simulink model "case2"  (R2024b)
settings: Solver=FixedStepAuto  StartTime=0  StopTime=1  FixedStep=1e-7  RelTol=1e-3
values from neighbouring files (symbols this model uses):
  SG_D_1_D = 0.01056    [IEEE9_case_parameters.m]    (also in case1_parameters.m; case2_parameters.m; case3_parameters.m; case4_parameters.m)
  SG_D_1_EnableSaturation = 0    [IEEE9_case_parameters.m]    (also in case1_parameters.m; case2_parameters.m; case3_parameters.m; case4_parameters.m)
  SG_D_1_f0 = 60    [IEEE9_case_parameters.m]    (also in case1_parameters.m; case2_parameters.m; case3_parameters.m; case4_parameters.m)
  SG_D_1_H = 7.5    [IEEE9_case_parameters.m]    (also in case1_parameters.m; case2_parameters.m; case3_parameters.m; case4_parameters.m)
  SG_D_1_K_A = 20    [IEEE9_case_parameters.m]    (also in case1_parameters.m; case2_parameters.m; case3_parameters.m; case4_parameters.m)
  SG_D_1_K_E = 1.000000e+1    (= 10)    [IEEE9_case_parameters.m]    (also in case1_parameters.m; case2_parameters.m; case3_parameters.m; case4_parameters.m)
  SG_D_1_K_F = 2.363    [IEEE9_case_parameters.m]    (also in case1_parameters.m; case2_parameters.m; case3_parameters.m; case4_parameters.m)
  SG_D_1_K_s = 0.5    [IEEE9_case_parameters.m]    (also in case1_parameters.m = 5; case2_parameters.m = 5; case3_parameters.m = 5; case4_parameters.m = 5)
  SG_D_1_R_a = 0.001088    [IEEE9_case_parameters.m]    (also in case1_parameters.m; case2_parameters.m; case3_parameters.m; case4_parameters.m)
  SG_D_1_S_A = 1    [IEEE9_case_parameters.m]    (also in case1_parameters.m; case2_parameters.m; case3_parameters.m; case4_parameters.m)
  SG_D_1_S_B = 0.103    [IEEE9_case_parameters.m]    (also in case1_parameters.m; case2_parameters.m; case3_parameters.m; case4_parameters.m)
  SG_D_1_S_N = 10.659857    [IEEE9_case_parameters.m]    (also in case1_parameters.m; case2_parameters.m; case3_parameters.m; case4_parameters.m)
  SG_D_1_SpeedPara = 200    [IEEE9_case_parameters.m]    (also in case1_parameters.m; case2_parameters.m; case3_parameters.m; case4_parameters.m)
  SG_D_1_T_0 = 0.720173    [IEEE9_case_parameters.m]    (also in case1_parameters.m = 0.755522; case2_parameters.m = 0.808931; case3_parameters.m = 0.869402; case4_parameters.m = 0.729316)
  SG_D_1_T_1 = 0.3    [IEEE9_case_parameters.m]    (also in case1_parameters.m; case2_parameters.m; case3_parameters.m; case4_parameters.m)
  SG_D_1_T_2 = 0.05    [IEEE9_case_parameters.m]    (also in case1_parameters.m; case2_parameters.m; case3_parameters.m; case4_parameters.m)
  SG_D_1_T_3 = 0.02    [IEEE9_case_parameters.m]    (also in case1_parameters.m; case2_parameters.m; case3_parameters.m; case4_parameters.m)
  SG_D_1_T_4 = 0.005    [IEEE9_case_parameters.m]    (also in case1_parameters.m; case2_parameters.m; case3_parameters.m; case4_parameters.m)
  SG_D_1_T_A = 0.02    [IEEE9_case_parameters.m]    (also in case1_parameters.m; case2_parameters.m; case3_parameters.m; case4_parameters.m)
  SG_D_1_T_dd = 8.000000e+0    (= 8)    [IEEE9_case_parameters.m]    (also in case1_parameters.m; case2_parameters.m; case3_parameters.m; case4_parameters.m)
  SG_D_1_T_ddd = 0.04    [IEEE9_case_parameters.m]    (also in case1_parameters.m; case2_parameters.m; case3_parameters.m; case4_parameters.m)
  SG_D_1_T_E = 0.314    [IEEE9_case_parameters.m]    (also in case1_parameters.m; case2_parameters.m; case3_parameters.m; case4_parameters.m)
  SG_D_1_T_F = 0.35    [IEEE9_case_parameters.m]    (also in case1_parameters.m; case2_parameters.m; case3_parameters.m; case4_parameters.m)
  SG_D_1_T_qd = 0.8    [IEEE9_case_parameters.m]    (also in case1_parameters.m; case2_parameters.m; case3_parameters.m; case4_parameters.m)
  SG_D_1_T_qdd = 0.02    [IEEE9_case_parameters.m]    (also in case1_parameters.m; case2_parameters.m; case3_parameters.m; case4_parameters.m)
  SG_D_1_T_speed = 0.1    [IEEE9_case_parameters.m]    (also in case1_parameters.m = 200; case2_parameters.m = 200; case3_parameters.m = 200; case4_parameters.m = 200)
  SG_D_1_T_w = 0.5    [IEEE9_case_parameters.m]    (also in case1_parameters.m; case2_parameters.m; case3_parameters.m; case4_parameters.m)
  SG_D_1_V_ref = 1.990276    [IEEE9_case_parameters.m]    (also in case1_parameters.m = 2.042296; case2_parameters.m = 2.051388; case3_parameters.m = 2.089584; case4_parameters.m = 2.01845)
  SG_D_1_w_ref = 376.991118    [IEEE9_case_parameters.m]    (also in case1_parameters.m; case2_parameters.m; case3_parameters.m; case4_parameters.m)
  SG_D_1_wb = 6.000000e+1    (= 60)    [IEEE9_case_parameters.m]    (also in case1_parameters.m; case2_parameters.m; case3_parameters.m; case4_parameters.m)
  SG_D_1_x_d = 1.9    [IEEE9_case_parameters.m]    (also in case1_parameters.m; case2_parameters.m; case3_parameters.m; case4_parameters.m)
  SG_D_1_x_dd = 0.302    [IEEE9_case_parameters.m]    (also in case1_parameters.m; case2_parameters.m; case3_parameters.m; case4_parameters.m)
  SG_D_1_x_ddd = 0.204    [IEEE9_case_parameters.m]    (also in case1_parameters.m; case2_parameters.m; case3_parameters.m; case4_parameters.m)
  SG_D_1_x_l = 0.05    [IEEE9_case_parameters.m]    (also in case1_parameters.m; case2_parameters.m; case3_parameters.m; case4_parameters.m)
  SG_D_1_x_q = 1.3    [IEEE9_case_parameters.m]    (also in case1_parameters.m; case2_parameters.m; case3_parameters.m; case4_parameters.m)
  SG_D_1_x_qd = 0.5    [IEEE9_case_parameters.m]    (also in case1_parameters.m; case2_parameters.m; case3_parameters.m; case4_parameters.m)
  SG_D_1_x_qdd = 0.3    [IEEE9_case_parameters.m]    (also in case1_parameters.m; case2_parameters.m; case3_parameters.m; case4_parameters.m)
  SG_D_2_D = 0.02    [IEEE9_case_parameters.m]    (also in case1_parameters.m; case2_parameters.m; case3_parameters.m; case4_parameters.m)
  SG_D_2_EnableSaturation = 0    [IEEE9_case_parameters.m]    (also in case1_parameters.m; case2_parameters.m; case3_parameters.m; case4_parameters.m)
  SG_D_2_f0 = 60    [IEEE9_case_parameters.m]    (also in case1_parameters.m; case2_parameters.m; case3_parameters.m; case4_parameters.m)
  SG_D_2_H = 8.000000e+0    (= 8)    [IEEE9_case_parameters.m]    (also in case1_parameters.m; case2_parameters.m; case3_parameters.m; case4_parameters.m)
  SG_D_2_K_A = 20    [IEEE9_case_parameters.m]    (also in case1_parameters.m; case2_parameters.m; case3_parameters.m; case4_parameters.m)
  SG_D_2_K_E = 1.000000e+1    (= 10)    [IEEE9_case_parameters.m]    (also in case1_parameters.m; case2_parameters.m; case3_parameters.m; case4_parameters.m)
  SG_D_2_K_F = 2.363    [IEEE9_case_parameters.m]    (also in case1_parameters.m; case2_parameters.m; case3_parameters.m; case4_parameters.m)
  SG_D_2_K_s = 0.5    [IEEE9_case_parameters.m]    (also in case1_parameters.m = 4; case2_parameters.m = 4; case3_parameters.m = 4; case4_parameters.m = 4)
  SG_D_2_R_a = 0.001088    [IEEE9_case_parameters.m]    (also in case1_parameters.m; case2_parameters.m; case3_parameters.m; case4_parameters.m)
  SG_D_2_S_A = 1    [IEEE9_case_parameters.m]    (also in case1_parameters.m; case2_parameters.m; case3_parameters.m; case4_parameters.m)
  SG_D_2_S_B = 0.103    [IEEE9_case_parameters.m]    (also in case1_parameters.m; case2_parameters.m; case3_parameters.m; case4_parameters.m)
  SG_D_2_S_N = 10.659857    [IEEE9_case_parameters.m]    (also in case1_parameters.m; case2_parameters.m; case3_parameters.m; case4_parameters.m)
  SG_D_2_SpeedPara = 200    [IEEE9_case_parameters.m]    (also in case1_parameters.m; case2_parameters.m; case3_parameters.m; case4_parameters.m)
  SG_D_2_T_0 = 1.632913    [IEEE9_case_parameters.m]    (also in case1_parameters.m = 1.632925; case2_parameters.m = 1.632915; case3_parameters.m = 1.632914; case4_parameters.m = 1.632927)
  SG_D_2_T_1 = 0.2    [IEEE9_case_parameters.m]    (also in case1_parameters.m; case2_parameters.m; case3_parameters.m; case4_parameters.m)
  SG_D_2_T_2 = 0.05    [IEEE9_case_parameters.m]    (also in case1_parameters.m; case2_parameters.m; case3_parameters.m; case4_parameters.m)
  SG_D_2_T_3 = 0.02    [IEEE9_case_parameters.m]    (also in case1_parameters.m; case2_parameters.m; case3_parameters.m; case4_parameters.m)
  SG_D_2_T_4 = 0.005    [IEEE9_case_parameters.m]    (also in case1_parameters.m; case2_parameters.m; case3_parameters.m; case4_parameters.m)
  SG_D_2_T_A = 0.02    [IEEE9_case_parameters.m]    (also in case1_parameters.m; case2_parameters.m; case3_parameters.m; case4_parameters.m)
  SG_D_2_T_dd = 7.9    [IEEE9_case_parameters.m]    (also in case1_parameters.m; case2_parameters.m; case3_parameters.m; case4_parameters.m)
  SG_D_2_T_ddd = 0.04    [IEEE9_case_parameters.m]    (also in case1_parameters.m; case2_parameters.m; case3_parameters.m; case4_parameters.m)
  SG_D_2_T_E = 0.314    [IEEE9_case_parameters.m]    (also in case1_parameters.m; case2_parameters.m; case3_parameters.m; case4_parameters.m)
  SG_D_2_T_F = 0.35    [IEEE9_case_parameters.m]    (also in case1_parameters.m; case2_parameters.m; case3_parameters.m; case4_parameters.m)
  SG_D_2_T_qd = 0.8    [IEEE9_case_parameters.m]    (also in case1_parameters.m; case2_parameters.m; case3_parameters.m; case4_parameters.m)
  SG_D_2_T_qdd = 0.015    [IEEE9_case_parameters.m]    (also in case1_parameters.m; case2_parameters.m; case3_parameters.m; case4_parameters.m)
  SG_D_2_T_speed = 0.1    [IEEE9_case_parameters.m]    (also in case1_parameters.m = 150; case2_parameters.m = 150; case3_parameters.m = 150; case4_parameters.m = 150)
  SG_D_2_T_w = 0.35    [IEEE9_case_parameters.m]    (also in case1_parameters.m; case2_parameters.m; case3_parameters.m; case4_parameters.m)
  SG_D_2_V_ref = 2.58547    [IEEE9_case_parameters.m]    (also in case1_parameters.m = 2.597896; case2_parameters.m = 2.587136; case3_parameters.m = 2.586042; case4_parameters.m = 2.599679)
  SG_D_2_w_ref = 376.991118    [IEEE9_case_parameters.m]    (also in case1_parameters.m; case2_parameters.m; case3_parameters.m; case4_parameters.m)
  SG_D_2_wb = 6.000000e+1    (= 60)    [IEEE9_case_parameters.m]    (also in case1_parameters.m; case2_parameters.m; case3_parameters.m; case4_parameters.m)
  SG_D_2_x_d = 1.8    [IEEE9_case_parameters.m]    (also in case1_parameters.m; case2_parameters.m; case3_parameters.m; case4_parameters.m)
  SG_D_2_x_dd = 0.302    [IEEE9_case_parameters.m]    (also in case1_parameters.m; case2_parameters.m; case3_parameters.m; case4_parameters.m)
  SG_D_2_x_ddd = 0.204    [IEEE9_case_parameters.m]    (also in case1_parameters.m; case2_parameters.m; case3_parameters.m; case4_parameters.m)
  SG_D_2_x_l = 0.05    [IEEE9_case_parameters.m]    (also in case1_parameters.m; case2_parameters.m; case3_parameters.m; case4_parameters.m)
  SG_D_2_x_q = 1.25    [IEEE9_case_parameters.m]    (also in case1_parameters.m; case2_parameters.m; case3_parameters.m; case4_parameters.m)
  SG_D_2_x_qd = 0.5    [IEEE9_case_parameters.m]    (also in case1_parameters.m; case2_parameters.m; case3_parameters.m; case4_parameters.m)
  SG_D_2_x_qdd = 0.3    [IEEE9_case_parameters.m]    (also in case1_parameters.m; case2_parameters.m; case3_parameters.m; case4_parameters.m)
  SG_D_3_D = 0.02    [IEEE9_case_parameters.m]    (also in case1_parameters.m; case2_parameters.m; case3_parameters.m; case4_parameters.m)
  SG_D_3_EnableSaturation = 0    [IEEE9_case_parameters.m]    (also in case1_parameters.m; case2_parameters.m; case3_parameters.m; case4_parameters.m)
  SG_D_3_f0 = 60    [IEEE9_case_parameters.m]    (also in case1_parameters.m; case2_parameters.m; case3_parameters.m; case4_parameters.m)
  SG_D_3_H = 7.7    [IEEE9_case_parameters.m]    (also in case1_parameters.m; case2_parameters.m; case3_parameters.m; case4_parameters.m)
  SG_D_3_K_A = 20    [IEEE9_case_parameters.m]    (also in case1_parameters.m; case2_parameters.m; case3_parameters.m; case4_parameters.m)
  SG_D_3_K_E = 1.000000e+1    (= 10)    [IEEE9_case_parameters.m]    (also in case1_parameters.m; case2_parameters.m; case3_parameters.m; case4_parameters.m)
  SG_D_3_K_F = 2.363    [IEEE9_case_parameters.m]    (also in case1_parameters.m; case2_parameters.m; case3_parameters.m; case4_parameters.m)
  SG_D_3_K_s = 0.2    [IEEE9_case_parameters.m]    (also in case1_parameters.m = 2; case2_parameters.m = 2; case3_parameters.m = 2; case4_parameters.m = 2)
  SG_D_3_R_a = 0.001088    [IEEE9_case_parameters.m]    (also in case1_parameters.m; case2_parameters.m; case3_parameters.m; case4_parameters.m)
  SG_D_3_S_A = 1    [IEEE9_case_parameters.m]    (also in case1_parameters.m; case2_parameters.m; case3_parameters.m; case4_parameters.m)
  SG_D_3_S_B = 0.103    [IEEE9_case_parameters.m]    (also in case1_parameters.m; case2_parameters.m; case3_parameters.m; case4_parameters.m)
  SG_D_3_S_N = 10.659857    [IEEE9_case_parameters.m]    (also in case1_parameters.m; case2_parameters.m; case3_parameters.m; case4_parameters.m)
  SG_D_3_SpeedPara = 200    [IEEE9_case_parameters.m]    (also in case1_parameters.m; case2_parameters.m; case3_parameters.m; case4_parameters.m)
  SG_D_3_T_0 = 0.850788    [IEEE9_case_parameters.m]    (also in case1_parameters.m = 0.850786; case2_parameters.m = 0.850787; case3_parameters.m; case4_parameters.m = 0.850786)
  SG_D_3_T_1 = 0.2    [IEEE9_case_parameters.m]    (also in case1_parameters.m; case2_parameters.m; case3_parameters.m; case4_parameters.m)
  SG_D_3_T_2 = 0.05    [IEEE9_case_parameters.m]    (also in case1_parameters.m; case2_parameters.m; case3_parameters.m; case4_parameters.m)
  SG_D_3_T_3 = 0.02    [IEEE9_case_parameters.m]    (also in case1_parameters.m; case2_parameters.m; case3_parameters.m; case4_parameters.m)
  SG_D_3_T_4 = 0.005    [IEEE9_case_parameters.m]    (also in case1_parameters.m; case2_parameters.m; case3_parameters.m; case4_parameters.m)
  SG_D_3_T_A = 0.02    [IEEE9_case_parameters.m]    (also in case1_parameters.m; case2_parameters.m; case3_parameters.m; case4_parameters.m)
  SG_D_3_T_dd = 8.1    [IEEE9_case_parameters.m]    (also in case1_parameters.m; case2_parameters.m; case3_parameters.m; case4_parameters.m)
  SG_D_3_T_ddd = 0.04    [IEEE9_case_parameters.m]    (also in case1_parameters.m; case2_parameters.m; case3_parameters.m; case4_parameters.m)
  SG_D_3_T_E = 0.314    [IEEE9_case_parameters.m]    (also in case1_parameters.m; case2_parameters.m; case3_parameters.m; case4_parameters.m)
  SG_D_3_T_F = 0.35    [IEEE9_case_parameters.m]    (also in case1_parameters.m; case2_parameters.m; case3_parameters.m; case4_parameters.m)
  SG_D_3_T_qd = 0.8    [IEEE9_case_parameters.m]    (also in case1_parameters.m; case2_parameters.m; case3_parameters.m; case4_parameters.m)
  SG_D_3_T_qdd = 0.015    [IEEE9_case_parameters.m]    (also in case1_parameters.m; case2_parameters.m; case3_parameters.m; case4_parameters.m)
  SG_D_3_T_speed = 0.1    [IEEE9_case_parameters.m]    (also in case1_parameters.m = 180; case2_parameters.m = 180; case3_parameters.m = 180; case4_parameters.m = 180)
  SG_D_3_T_w = 0.4    [IEEE9_case_parameters.m]    (also in case1_parameters.m; case2_parameters.m; case3_parameters.m; case4_parameters.m)
  SG_D_3_V_ref = 1.892727    [IEEE9_case_parameters.m]    (also in case1_parameters.m = 1.906439; case2_parameters.m = 1.895535; case3_parameters.m = 1.892105; case4_parameters.m = 1.906598)
  SG_D_3_w_ref = 376.991118    [IEEE9_case_parameters.m]    (also in case1_parameters.m; case2_parameters.m; case3_parameters.m; case4_parameters.m)
  SG_D_3_wb = 6.000000e+1    (= 60)    [IEEE9_case_parameters.m]    (also in case1_parameters.m; case2_parameters.m; case3_parameters.m; case4_parameters.m)
  SG_D_3_x_d = 1.85    [IEEE9_case_parameters.m]    (also in case1_parameters.m; case2_parameters.m; case3_parameters.m; case4_parameters.m)
  SG_D_3_x_dd = 0.302    [IEEE9_case_parameters.m]    (also in case1_parameters.m; case2_parameters.m; case3_parameters.m; case4_parameters.m)
  SG_D_3_x_ddd = 0.204    [IEEE9_case_parameters.m]    (also in case1_parameters.m; case2_parameters.m; case3_parameters.m; case4_parameters.m)
  SG_D_3_x_l = 0.05    [IEEE9_case_parameters.m]    (also in case1_parameters.m; case2_parameters.m; case3_parameters.m; case4_parameters.m)
  SG_D_3_x_q = 1.2    [IEEE9_case_parameters.m]    (also in case1_parameters.m; case2_parameters.m; case3_parameters.m; case4_parameters.m)
  SG_D_3_x_qd = 0.5    [IEEE9_case_parameters.m]    (also in case1_parameters.m; case2_parameters.m; case3_parameters.m; case4_parameters.m)
  SG_D_3_x_qdd = 0.3    [IEEE9_case_parameters.m]    (also in case1_parameters.m; case2_parameters.m; case3_parameters.m; case4_parameters.m)
(part 10 of 12)

== system case2/SG_D_3/d_R_f_SG_D_3_block ==
  note: d_R_f_SG_D_3 in case2
      | $-\frac{R_{f,\mathrm{SG},D,3}-\frac{E_{\mathrm{fd},\mathrm{SG},D,3}\,K_{F}}{T_{F}}}{T_{F}}$
      | Automatically generated on 2025-10-31 18:56:03 .
  State_E_fd_SG_D_3_decea : Inport
  State_R_f_SG_D_3_e823d : Inport  Port=2
  Constant_K_F_23a0b : Constant  Value=K_F
  Constant_T_F_23cea : Constant  Value=T_F
  Constant_T_F_8318a : Constant  Value=T_F
  Divide_03d04 : Product  Inputs=*/
  Divide_99c86 : Product  Inputs=*/
  Product_79fc5 : Product
  Subtract_db161 : Sum  Inputs=+-
  Blockout_d_R_f_SG_D_3_2f717 : Outport
  wires:
  State_E_fd_SG_D_3_decea/1 -> Product_79fc5/1
  Constant_T_F_8318a/1 -> Divide_99c86/2
  Constant_K_F_23a0b/1 -> Product_79fc5/2
  Product_79fc5/1 -> Divide_99c86/1
  Divide_99c86/1 -> Subtract_db161/1
  State_R_f_SG_D_3_e823d/1 -> Subtract_db161/2
  Subtract_db161/1 -> Divide_03d04/1
  Constant_T_F_23cea/1 -> Divide_03d04/2
  Divide_03d04/1 -> Blockout_d_R_f_SG_D_3_2f717/1

== system case2/SG_D_3/d_T_m_SG_D_3_block ==
  note: d_T_m_SG_D_3 in case2
      | $-\frac{T_{m,\mathrm{SG},D,3}-T_{0}+\frac{\mathrm{SpeedPara}\,\left(w_{\mathrm{SG},D,3}-w_{\mathrm{ref}}\right)}{2\,f_{0}\,\pi }}{T_{\mathrm{speed}}}$
      | Automatically generated on 2025-10-31 18:55:54 .
  State_w_SG_D_3_ad955 : Inport
  State_T_m_SG_D_3_dcae6 : Inport  Port=2
  Add_1559f : Sum
  Add_c16dd : Sum
  Constant_-1_b8cee : Constant  Value=-1
  Constant_2.0_46722 : Constant  Value=2.0
  Constant_SpeedPara_f1b9d : Constant  Value=SpeedPara
  Constant_T_0_ab028 : Constant  Value=T_0
  Constant_T_speed_635f7 : Constant  Value=T_speed
  Constant_f0_5bcf7 : Constant  Value=f0
  Constant_pi_42e70 : Constant  Value=pi
  Constant_w_ref_c3ceb : Constant  Value=w_ref
  Divide_6bed0 : Product  Inputs=*/
  Divide_af97e : Product  Inputs=*/
  Product_4a7b1 : Product
  Product_d472e : Product
  Product_e3a05 : Product
  Product_e8c78 : Product
  Subtract_c2881 : Sum  Inputs=+-
  Blockout_d_T_m_SG_D_3_4be0a : Outport
  wires:
  Constant_SpeedPara_f1b9d/1 -> Product_d472e/1
  Constant_-1_b8cee/1 -> Product_e8c78/1
  Constant_w_ref_c3ceb/1 -> Add_c16dd/2
  State_w_SG_D_3_ad955/1 -> Product_e8c78/2
  Constant_2.0_46722/1 -> Product_4a7b1/1
  Product_e8c78/1 -> Add_c16dd/1
  Constant_pi_42e70/1 -> Product_4a7b1/2
  Add_c16dd/1 -> Product_d472e/2
  Product_4a7b1/1 -> Product_e3a05/1
  Constant_f0_5bcf7/1 -> Product_e3a05/2
  Product_d472e/1 -> Divide_af97e/1
  Product_e3a05/1 -> Divide_af97e/2
  Divide_af97e/1 -> Add_1559f/1
  Constant_T_0_ab028/1 -> Add_1559f/2
  Add_1559f/1 -> Subtract_c2881/1
  State_T_m_SG_D_3_dcae6/1 -> Subtract_c2881/2
  Subtract_c2881/1 -> Divide_6bed0/1
  Constant_T_speed_635f7/1 -> Divide_6bed0/2
  Divide_6bed0/1 -> Blockout_d_T_m_SG_D_3_4be0a/1

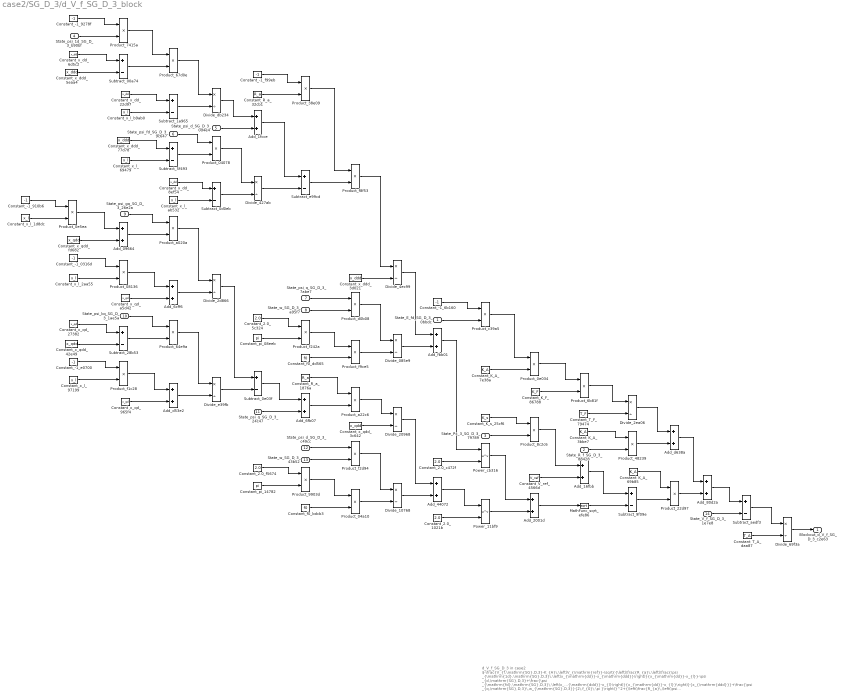
== system case2/SG_D_3/d_V_f_SG_D_3_block ==
  note: d_V_f_SG_D_3 in case2
      | $-\frac{V_{f,\mathrm{SG},D,3}-K_{A}\,\left(V_{\mathrm{ref}}-\sqrt{{\left(\frac{R_{a}\,\left(\frac{\psi _{\mathrm{1d},\mathrm{SG},D,3}\,\left(x_{\mathrm{dd}}-x_{\mathrm{ddd}}\right)}{x_{\mathrm{dd}}-x_{l}}-\psi _{d,\mathrm{SG},D,3}+\frac{\psi _{\mathrm{fd},\mathrm{SG},D,3}\,\left(x_{\mathrm{ddd}}-x_{l}\right)}{x_{\mathrm{dd}}-x_{l}}\right)}{x_{\mathrm{ddd}}}+\frac{\psi _{q,\mathrm{SG},D,3}\,w_{\mathrm{SG},D,3}}{2\,f_{0}\,\pi }\right)}^2+{\left(\frac{R_{a}\,\left(\psi _{q,\mathrm{SG},D,3}+\frac{\psi _{\mathrm{gq},\mathrm{SG},D,3}\,\left(x_{l}-x_{\mathrm{qdd}}\right)}{x_{l}-x_{\mathrm{qd}}}+\frac{\psi _{\mathrm{kq},\mathrm{SG},D,3}\,\left(x_{\mathrm{qd}}-x_{\mathrm{qdd}}\right)}{x_{l}-x_{\mathrm{qd}}}\right)}{x_{\mathrm{qdd}}}+\frac{\psi _{d,\mathrm{SG},D,3}\,w_{\mathrm{SG},D,3}}{2\,f_{0}\,\pi }\right)}^2}+K_{s}\,\mathrm{Px}_{3,\mathrm{SG},D,3}\right)-K_{A}\,R_{f,\mathrm{SG},D,3}+\frac{E_{\mathrm{fd},\mathrm{SG},D,3}\,K_{A}\,K_{F}}{T_{F}}}{T_{A}}$
      | Automatically generated on 2025-10-31 18:56:01 .
  State_E_fd_SG_D_3_0bbdc : Inport
  State_R_f_SG_D_3_88428 : Inport  Port=2
  State_Px_3_SG_D_3_79789 : Inport  Port=3
  State_psi_1d_SG_D_3_b90bf : Inport  Port=4
  State_psi_d_SG_D_3_0d4e4 : Inport  Port=5
  State_psi_fd_SG_D_3_9c647 : Inport  Port=6
  State_psi_q_SG_D_3_7abe7 : Inport  Port=7
  State_w_SG_D_3_a95f7 : Inport  Port=8
  State_psi_gq_SG_D_3_26e2a : Inport  Port=9
  State_psi_kq_SG_D_3_1ae5a : Inport  Port=10
  State_psi_q_SG_D_3_24c47 : Inport  Port=11
  State_psi_d_SG_D_3_c49cc : Inport  Port=12
  State_w_SG_D_3_43b52 : Inport  Port=13
  State_V_f_SG_D_3_1e7e8 : Inport  Port=14
  Add_09664 : Sum
  Add_16fbb : Sum
  Add_1fcce : Sum
  Add_2001d : Sum
  Add_44072 : Sum
  Add_6cff6 : Sum
  Add_6fb07 : Sum
  Add_80d2a : Sum
  Add_d53e2 : Sum
  Add_d638a : Sum
  Add_fbb01 : Sum
  Constant_-1_0316d : Constant  Value=-1
  Constant_-1_6b160 : Constant  Value=-1
  Constant_-1_910b6 : Constant  Value=-1
  Constant_-1_9278f : Constant  Value=-1
  Constant_-1_e0700 : Constant  Value=-1
  Constant_-1_f99eb : Constant  Value=-1
  Constant_2.0_1021b : Constant  Value=2.0
  Constant_2.0_5c324 : Constant  Value=2.0
  Constant_2.0_c472f : Constant  Value=2.0
  Constant_2.0_f5674 : Constant  Value=2.0
  Constant_K_A_3bbe7 : Constant  Value=K_A
  Constant_K_A_69b85 : Constant  Value=K_A
  Constant_K_A_7e38a : Constant  Value=K_A
  Constant_K_F_86788 : Constant  Value=K_F
  Constant_K_s_25cf6 : Constant  Value=K_s
  Constant_R_a_1876a : Constant  Value=R_a
  Constant_R_a_32cb1 : Constant  Value=R_a
  Constant_T_A_daa87 : Constant  Value=T_A
  Constant_T_F_79474 : Constant  Value=T_F
  Constant_V_ref_4566d : Constant  Value=V_ref
  Constant_f0_bdcb3 : Constant  Value=f0
  Constant_f0_dd565 : Constant  Value=f0
  Constant_pi_08eeb : Constant  Value=pi
  Constant_pi_14782 : Constant  Value=pi
  Constant_x_dd_22d97 : Constant  Value=x_dd
  Constant_x_dd_6d5c2 : Constant  Value=x_dd
  Constant_x_dd_8ef54 : Constant  Value=x_dd
  Constant_x_ddd_3d021 : Constant  Value=x_ddd
  Constant_x_ddd_5eaa4 : Constant  Value=x_ddd
  Constant_x_ddd_77d78 : Constant  Value=x_ddd
  Constant_x_l_1d8dc : Constant  Value=x_l
  Constant_x_l_2aa55 : Constant  Value=x_l
  Constant_x_l_69479 : Constant  Value=x_l
  Constant_x_l_97199 : Constant  Value=x_l
  Constant_x_l_ab532 : Constant  Value=x_l
  Constant_x_l_b9ab0 : Constant  Value=x_l
  Constant_x_qd_27382 : Constant  Value=x_qd
  Constant_x_qd_965f4 : Constant  Value=x_qd
  Constant_x_qd_a5d42 : Constant  Value=x_qd
  Constant_x_qdd_3c642 : Constant  Value=x_qdd
  Constant_x_qdd_42e49 : Constant  Value=x_qdd
  Constant_x_qdd_fd682 : Constant  Value=x_qdd
  Divide_085e9 : Product  Inputs=*/
  Divide_10768 : Product  Inputs=*/
  Divide_20968 : Product  Inputs=*/
  Divide_2d866 : Product  Inputs=*/
  Divide_2ea06 : Product  Inputs=*/
  Divide_427ab : Product  Inputs=*/
  Divide_4ec99 : Product  Inputs=*/
  Divide_69f3a : Product  Inputs=*/
  Divide_db234 : Product  Inputs=*/
  Divide_e39fb : Product  Inputs=*/
  MathFunc_sqrt_efe86 : Sqrt
  Power_11bf9 : Math  Operator=pow
  Power_cb316 : Math  Operator=pow
  Product_04078 : Product
  Product_04a10 : Product
  Product_08136 : Product
  Product_0e034 : Product
  Product_0e5ea : Product
  Product_22d97 : Product
  Product_38e09 : Product
  Product_48239 : Product
  Product_64e9a : Product
  Product_67d0e : Product
  Product_6b81f : Product
  Product_7415a : Product
  Product_8c2c6 : Product
  Product_9903d : Product
  Product_a020a : Product
  Product_a22c6 : Product
  Product_c39a5 : Product
  Product_d0b08 : Product
  Product_f1c28 : Product
  Product_f242a : Product
  Product_f2d94 : Product
  Product_f8f53 : Product
  Product_f9ce5 : Product
  Subtract_00a74 : Sum  Inputs=+-
  Subtract_0d0eb : Sum  Inputs=+-
  Subtract_0e03f : Sum  Inputs=+-
  Subtract_1a965 : Sum  Inputs=+-
  Subtract_28b53 : Sum  Inputs=+-
  Subtract_5f493 : Sum  Inputs=+-
  Subtract_9f09e : Sum  Inputs=+-
  Subtract_aedf3 : Sum  Inputs=+-
  Subtract_e99cd : Sum  Inputs=+-
  Blockout_d_V_f_SG_D_3_c2e63 : Outport
  wires:
  Constant_K_A_3bbe7/1 -> Product_48239/1
  Constant_-1_910b6/1 -> Product_0e5ea/1
  Subtract_5f493/1 -> Product_04078/2
  Constant_x_l_1d8dc/1 -> Product_0e5ea/2
  Divide_10768/1 -> Add_44072/2
  Constant_-1_9278f/1 -> Product_7415a/1
  State_psi_1d_SG_D_3_b90bf/1 -> Product_7415a/2
  Constant_x_dd_6d5c2/1 -> Subtract_00a74/1
  Divide_427ab/1 -> Subtract_e99cd/2
  Product_0e5ea/1 -> Add_09664/1
  Constant_x_qdd_fd682/1 -> Add_09664/2
  Constant_x_ddd_5eaa4/1 -> Subtract_00a74/2
  Constant_2.0_1021b/1 -> Power_11bf9/2
  Constant_-1_0316d/1 -> Product_08136/1
  Divide_2d866/1 -> Subtract_0e03f/1
  Subtract_1a965/1 -> Divide_db234/2
  Constant_x_l_2aa55/1 -> Product_08136/2
  Constant_x_qd_27382/1 -> Subtract_28b53/1
  State_w_SG_D_3_a95f7/1 -> Product_d0b08/2
  Constant_x_qdd_42e49/1 -> Subtract_28b53/2
  Constant_2.0_5c324/1 -> Product_f242a/1
  Constant_-1_e0700/1 -> Product_f1c28/1
  Constant_pi_08eeb/1 -> Product_f242a/2
  Add_1fcce/1 -> Subtract_e99cd/1
  Constant_x_l_97199/1 -> Product_f1c28/2
  Product_7415a/1 -> Product_67d0e/1
  Subtract_00a74/1 -> Product_67d0e/2
  Constant_2.0_f5674/1 -> Product_9903d/1
  Constant_x_dd_22d97/1 -> Subtract_1a965/1
  Constant_pi_14782/1 -> Product_9903d/2
  Constant_x_l_b9ab0/1 -> Subtract_1a965/2
  Constant_x_ddd_77d78/1 -> Subtract_5f493/1
  Constant_x_l_69479/1 -> Subtract_5f493/2
  State_psi_gq_SG_D_3_26e2a/1 -> Product_a020a/1
  Constant_x_l_ab532/1 -> Subtract_0d0eb/2
  Add_09664/1 -> Product_a020a/2
  Product_08136/1 -> Add_6cff6/1
  Product_a020a/1 -> Divide_2d866/1
  Constant_x_qd_a5d42/1 -> Add_6cff6/2
  State_psi_kq_SG_D_3_1ae5a/1 -> Product_64e9a/1
  State_psi_q_SG_D_3_7abe7/1 -> Product_d0b08/1
  Add_fbb01/1 -> Power_cb316/1
  Subtract_28b53/1 -> Product_64e9a/2
  Constant_f0_dd565/1 -> Product_f9ce5/2
  Product_f242a/1 -> Product_f9ce5/1
  Constant_x_qd_965f4/1 -> Add_d53e2/2
  Product_f1c28/1 -> Add_d53e2/1
  Product_67d0e/1 -> Divide_db234/1
  State_psi_fd_SG_D_3_9c647/1 -> Product_04078/1
  Constant_x_dd_8ef54/1 -> Subtract_0d0eb/1
  Add_6cff6/1 -> Divide_2d866/2
  Add_2001d/1 -> MathFunc_sqrt_efe86/1
  Product_64e9a/1 -> Divide_e39fb/1
  Add_d53e2/1 -> Divide_e39fb/2
  Product_38e09/1 -> Product_f8f53/1
  Divide_db234/1 -> Add_1fcce/1
  Add_16fbb/1 -> Subtract_9f09e/1
  State_psi_d_SG_D_3_0d4e4/1 -> Add_1fcce/2
  Product_04078/1 -> Divide_427ab/1
  Subtract_0d0eb/1 -> Divide_427ab/2
  MathFunc_sqrt_efe86/1 -> Subtract_9f09e/2
  Divide_e39fb/1 -> Subtract_0e03f/2
  Constant_-1_f99eb/1 -> Product_38e09/1
  Constant_R_a_32cb1/1 -> Product_38e09/2
  Subtract_0e03f/1 -> Add_6fb07/1
  State_psi_q_SG_D_3_24c47/1 -> Add_6fb07/2
  Subtract_e99cd/1 -> Product_f8f53/2
  Constant_R_a_1876a/1 -> Product_a22c6/1
  Add_6fb07/1 -> Product_a22c6/2
  State_psi_d_SG_D_3_c49cc/1 -> Product_f2d94/1
  State_w_SG_D_3_43b52/1 -> Product_f2d94/2
  Product_9903d/1 -> Product_04a10/1
  Constant_f0_bdcb3/1 -> Product_04a10/2
  Product_f8f53/1 -> Divide_4ec99/1
  Constant_x_ddd_3d021/1 -> Divide_4ec99/2
  Product_d0b08/1 -> Divide_085e9/1
  Product_f9ce5/1 -> Divide_085e9/2
  Product_a22c6/1 -> Divide_20968/1
  Constant_x_qdd_3c642/1 -> Divide_20968/2
  Product_f2d94/1 -> Divide_10768/1
  Product_04a10/1 -> Divide_10768/2
  Divide_4ec99/1 -> Add_fbb01/1
  Divide_085e9/1 -> Add_fbb01/2
  Divide_20968/1 -> Add_44072/1
  Constant_-1_6b160/1 -> Product_c39a5/1
  State_E_fd_SG_D_3_0bbdc/1 -> Product_c39a5/2
  Constant_2.0_c472f/1 -> Power_cb316/2
  Add_44072/1 -> Power_11bf9/1
  Product_c39a5/1 -> Product_0e034/1
  Constant_K_A_7e38a/1 -> Product_0e034/2
  Constant_K_s_25cf6/1 -> Product_8c2c6/1
  State_Px_3_SG_D_3_79789/1 -> Product_8c2c6/2
  Power_cb316/1 -> Add_2001d/1
  Power_11bf9/1 -> Add_2001d/2
  Product_0e034/1 -> Product_6b81f/1
  Constant_K_F_86788/1 -> Product_6b81f/2
  Product_8c2c6/1 -> Add_16fbb/1
  Constant_V_ref_4566d/1 -> Add_16fbb/2
  Product_6b81f/1 -> Divide_2ea06/1
  Constant_T_F_79474/1 -> Divide_2ea06/2
  Add_80d2a/1 -> Subtract_aedf3/1
  State_R_f_SG_D_3_88428/1 -> Product_48239/2
  Divide_2ea06/1 -> Add_d638a/1
  Product_48239/1 -> Add_d638a/2
  Constant_K_A_69b85/1 -> Product_22d97/1
  Subtract_9f09e/1 -> Product_22d97/2
  Add_d638a/1 -> Add_80d2a/1
  Product_22d97/1 -> Add_80d2a/2
  State_V_f_SG_D_3_1e7e8/1 -> Subtract_aedf3/2
  Subtract_aedf3/1 -> Divide_69f3a/1
  Constant_T_A_daa87/1 -> Divide_69f3a/2
  Divide_69f3a/1 -> Blockout_d_V_f_SG_D_3_c2e63/1

== system case2/SG_D_3/d_psi_1d_SG_D_3_block ==
  note: d_psi_1d_SG_D_3 in case2
      | $-\frac{\psi _{\mathrm{1d},\mathrm{SG},D,3}-\psi _{\mathrm{fd},\mathrm{SG},D,3}+\frac{\left(x_{\mathrm{dd}}-x_{l}\right)\,\left(\frac{\psi _{\mathrm{1d},\mathrm{SG},D,3}\,\left(x_{\mathrm{dd}}-x_{\mathrm{ddd}}\right)}{x_{\mathrm{dd}}-x_{l}}-\psi _{d,\mathrm{SG},D,3}+\frac{\psi _{\mathrm{fd},\mathrm{SG},D,3}\,\left(x_{\mathrm{ddd}}-x_{l}\right)}{x_{\mathrm{dd}}-x_{l}}\right)}{x_{\mathrm{ddd}}}}{T_{\mathrm{ddd}}}$
      | Automatically generated on 2025-10-31 18:55:36 .
  State_psi_1d_SG_D_3_8bb29 : Inport
  State_psi_fd_SG_D_3_ea669 : Inport  Port=2
  State_psi_1d_SG_D_3_111f5 : Inport  Port=3
  State_psi_d_SG_D_3_a70b8 : Inport  Port=4
  State_psi_fd_SG_D_3_4d32c : Inport  Port=5
  Add_7d00f : Sum
  Add_81263 : Sum
  Add_ada25 : Sum
  Constant_-1_96bb3 : Constant  Value=-1
  Constant_-1_f7891 : Constant  Value=-1
  Constant_T_ddd_8c8cf : Constant  Value=T_ddd
  Constant_x_dd_4ba2d : Constant  Value=x_dd
  Constant_x_dd_6af1a : Constant  Value=x_dd
  Constant_x_dd_ccd5a : Constant  Value=x_dd
  Constant_x_dd_de68b : Constant  Value=x_dd
  Constant_x_ddd_04580 : Constant  Value=x_ddd
  Constant_x_ddd_2c30d : Constant  Value=x_ddd
  Constant_x_ddd_47fd2 : Constant  Value=x_ddd
  Constant_x_l_2d0d9 : Constant  Value=x_l
  Constant_x_l_72a0b : Constant  Value=x_l
  Constant_x_l_835f8 : Constant  Value=x_l
  Constant_x_l_ee439 : Constant  Value=x_l
  Divide_0a825 : Product  Inputs=*/
  Divide_a9b63 : Product  Inputs=*/
  Divide_f3971 : Product  Inputs=*/
  Divide_fb6ac : Product  Inputs=*/
  Product_006f4 : Product
  Product_7e149 : Product
  Product_ad8c0 : Product
  Product_c5d48 : Product
  Product_f72a3 : Product
  Subtract_3b828 : Sum  Inputs=+-
  Subtract_3c316 : Sum  Inputs=+-
  Subtract_9a59b : Sum  Inputs=+-
  Subtract_acf31 : Sum  Inputs=+-
  Subtract_d1b34 : Sum  Inputs=+-
  Subtract_e1ee3 : Sum  Inputs=+-
  Blockout_d_psi_1d_SG_D_3_f73a2 : Outport
  wires:
  Divide_fb6ac/1 -> Add_81263/1
  Subtract_3c316/1 -> Product_f72a3/2
  Constant_-1_f7891/1 -> Product_c5d48/1
  Constant_x_dd_de68b/1 -> Subtract_9a59b/1
  State_psi_1d_SG_D_3_111f5/1 -> Product_c5d48/2
  Product_c5d48/1 -> Product_f72a3/1
  Constant_x_dd_4ba2d/1 -> Subtract_3c316/1
  Constant_x_ddd_04580/1 -> Subtract_3c316/2
  Constant_x_l_72a0b/1 -> Subtract_9a59b/2
  Constant_x_ddd_47fd2/1 -> Subtract_e1ee3/1
  Divide_0a825/1 -> Blockout_d_psi_1d_SG_D_3_f73a2/1
  Constant_x_l_ee439/1 -> Subtract_e1ee3/2
  Product_f72a3/1 -> Divide_fb6ac/1
  Subtract_9a59b/1 -> Divide_fb6ac/2
  State_psi_fd_SG_D_3_4d32c/1 -> Product_006f4/1
  Subtract_e1ee3/1 -> Product_006f4/2
  Constant_x_dd_ccd5a/1 -> Subtract_acf31/1
  Constant_x_l_835f8/1 -> Subtract_acf31/2
  State_psi_d_SG_D_3_a70b8/1 -> Add_81263/2
  Product_006f4/1 -> Divide_a9b63/1
  Subtract_acf31/1 -> Divide_a9b63/2
  Constant_x_dd_6af1a/1 -> Subtract_d1b34/1
  Constant_x_l_2d0d9/1 -> Subtract_d1b34/2
  Add_81263/1 -> Subtract_3b828/1
  Divide_a9b63/1 -> Subtract_3b828/2
  Constant_-1_96bb3/1 -> Product_ad8c0/1
  State_psi_1d_SG_D_3_8bb29/1 -> Product_ad8c0/2
  State_psi_fd_SG_D_3_ea669/1 -> Add_7d00f/2
  Subtract_d1b34/1 -> Product_7e149/1
  Subtract_3b828/1 -> Product_7e149/2
  Product_ad8c0/1 -> Add_7d00f/1
  Product_7e149/1 -> Divide_f3971/1
  Constant_x_ddd_2c30d/1 -> Divide_f3971/2
  Add_7d00f/1 -> Add_ada25/1
  Divide_f3971/1 -> Add_ada25/2
  Add_ada25/1 -> Divide_0a825/1
  Constant_T_ddd_8c8cf/1 -> Divide_0a825/2

== system case2/SG_D_3/d_psi_d_SG_D_3_block ==
  note: d_psi_d_SG_D_3 in case2
      | $2\,\pi \,f_{0}\,\left(v_{d,\mathrm{SG},D,3}\,\sin\left(\theta _{\mathrm{SG},D,3}\right)-v_{q,\mathrm{SG},D,3}\,\cos\left(\theta _{\mathrm{SG},D,3}\right)+\frac{R_{a}\,\left(\frac{\psi _{\mathrm{1d},\mathrm{SG},D,3}\,\left(x_{\mathrm{dd}}-x_{\mathrm{ddd}}\right)}{x_{\mathrm{dd}}-x_{l}}-\psi _{d,\mathrm{SG},D,3}+\frac{\psi _{\mathrm{fd},\mathrm{SG},D,3}\,\left(x_{\mathrm{ddd}}-x_{l}\right)}{x_{\mathrm{dd}}-x_{l}}\right)}{x_{\mathrm{ddd}}}+\frac{\psi _{q,\mathrm{SG},D,3}\,w_{\mathrm{SG},D,3}}{2\,f_{0}\,\pi }\right)$
      | Automatically generated on 2025-10-31 18:55:24 .
  State_psi_1d_SG_D_3_a4437 : Inport
  State_psi_d_SG_D_3_921ca : Inport  Port=2
  State_psi_fd_SG_D_3_c348d : Inport  Port=3
  Input_v_d_SG_D_3_4a6e0 : Inport  Port=4
  State_theta_SG_D_3_26889 : Inport  Port=5
  Input_v_q_SG_D_3_b307b : Inport  Port=6
  State_theta_SG_D_3_a755b : Inport  Port=7
  State_psi_q_SG_D_3_2a9ae : Inport  Port=8
  State_w_SG_D_3_819b4 : Inport  Port=9
  Add_52737 : Sum
  Add_b5873 : Sum
  Constant_-1_7d1d3 : Constant  Value=-1
  Constant_-2.0_b3201 : Constant  Value=-2.0
  Constant_2.0_44dfe : Constant  Value=2.0
  Constant_R_a_fca9e : Constant  Value=R_a
  Constant_f0_3ed91 : Constant  Value=f0
  Constant_f0_88d2b : Constant  Value=f0
  Constant_pi_0cbca : Constant  Value=pi
  Constant_pi_57084 : Constant  Value=pi
  Constant_x_dd_2eb8c : Constant  Value=x_dd
  Constant_x_dd_30135 : Constant  Value=x_dd
  Constant_x_dd_dee40 : Constant  Value=x_dd
  Constant_x_ddd_04a70 : Constant  Value=x_ddd
  Constant_x_ddd_814d4 : Constant  Value=x_ddd
  Constant_x_ddd_9593d : Constant  Value=x_ddd
  Constant_x_l_3d087 : Constant  Value=x_l
  Constant_x_l_bd87b : Constant  Value=x_l
  Constant_x_l_e7ee6 : Constant  Value=x_l
  Divide_0839e : Product  Inputs=*/
  Divide_384c5 : Product  Inputs=*/
  Divide_74f28 : Product  Inputs=*/
  Divide_76a4e : Product  Inputs=*/
  MathFunc_cos_de504 : Trigonometry  Operator=cos
  MathFunc_sin_964e7 : Trigonometry
  Product_0bbf3 : Product
  Product_3daeb : Product
  Product_55e5e : Product
  Product_5d5ba : Product
  Product_60192 : Product
  Product_630b1 : Product
  Product_65e05 : Product
  Product_a0510 : Product
  Product_bdb88 : Product
  Product_c572b : Product
  Product_d79da : Product
  Product_decc0 : Product
  Subtract_23be1 : Sum  Inputs=+-
  Subtract_4a561 : Sum  Inputs=+-
  Subtract_52ed6 : Sum  Inputs=+-
  Subtract_70482 : Sum  Inputs=+-
  Subtract_7d913 : Sum  Inputs=+-
  Subtract_c33ed : Sum  Inputs=+-
  Subtract_dcd4a : Sum  Inputs=+-
  Blockout_d_psi_d_SG_D_3_d08c6 : Outport
  wires:
  Constant_-1_7d1d3/1 -> Product_3daeb/1
  Constant_2.0_44dfe/1 -> Product_5d5ba/1
  Constant_x_dd_30135/1 -> Subtract_70482/1
  State_psi_1d_SG_D_3_a4437/1 -> Product_3daeb/2
  Constant_x_dd_dee40/1 -> Subtract_4a561/1
  Constant_pi_0cbca/1 -> Product_5d5ba/2
  Constant_x_ddd_9593d/1 -> Subtract_70482/2
  Product_3daeb/1 -> Product_bdb88/1
  Product_5d5ba/1 -> Product_a0510/1
  Subtract_70482/1 -> Product_bdb88/2
  Constant_-2.0_b3201/1 -> Product_0bbf3/1
  Constant_x_l_bd87b/1 -> Subtract_4a561/2
  Constant_x_ddd_04a70/1 -> Subtract_dcd4a/1
  Constant_pi_57084/1 -> Product_0bbf3/2
  Constant_x_l_3d087/1 -> Subtract_dcd4a/2
  Product_60192/1 -> Divide_74f28/1
  Product_bdb88/1 -> Divide_76a4e/1
  Subtract_4a561/1 -> Divide_76a4e/2
  State_psi_fd_SG_D_3_c348d/1 -> Product_c572b/1
  Subtract_dcd4a/1 -> Product_c572b/2
  Constant_x_dd_2eb8c/1 -> Subtract_52ed6/1
  Constant_x_l_e7ee6/1 -> Subtract_52ed6/2
  Divide_74f28/1 -> Subtract_c33ed/2
  Divide_76a4e/1 -> Add_b5873/1
  Subtract_7d913/1 -> Product_55e5e/2
  State_psi_d_SG_D_3_921ca/1 -> Add_b5873/2
  Product_c572b/1 -> Divide_0839e/1
  Subtract_52ed6/1 -> Divide_0839e/2
  Add_b5873/1 -> Subtract_7d913/1
  Divide_0839e/1 -> Subtract_7d913/2
  Product_65e05/1 -> Add_52737/2
  Constant_R_a_fca9e/1 -> Product_55e5e/1
  Product_d79da/1 -> Product_decc0/1
  State_theta_SG_D_3_26889/1 -> MathFunc_sin_964e7/1
  Product_55e5e/1 -> Divide_384c5/1
  Constant_x_ddd_814d4/1 -> Divide_384c5/2
  Input_v_d_SG_D_3_4a6e0/1 -> Product_630b1/1
  State_w_SG_D_3_819b4/1 -> Product_60192/2
  MathFunc_sin_964e7/1 -> Product_630b1/2
  State_theta_SG_D_3_a755b/1 -> MathFunc_cos_de504/1
  MathFunc_cos_de504/1 -> Product_65e05/2
  Divide_384c5/1 -> Subtract_23be1/1
  Product_630b1/1 -> Subtract_23be1/2
  Input_v_q_SG_D_3_b307b/1 -> Product_65e05/1
  State_psi_q_SG_D_3_2a9ae/1 -> Product_60192/1
  Constant_f0_3ed91/1 -> Product_a0510/2
  Subtract_23be1/1 -> Add_52737/1
  Product_a0510/1 -> Divide_74f28/2
  Product_0bbf3/1 -> Product_d79da/1
  Constant_f0_88d2b/1 -> Product_d79da/2
  Add_52737/1 -> Subtract_c33ed/1
  Subtract_c33ed/1 -> Product_decc0/2
  Product_decc0/1 -> Blockout_d_psi_d_SG_D_3_d08c6/1

== system case2/SG_D_3/d_psi_fd_SG_D_3_block ==
  note: d_psi_fd_SG_D_3 in case2
      | $-\frac{\psi _{\mathrm{fd},\mathrm{SG},D,3}-E_{\mathrm{fd},\mathrm{SG},D,3}+\left(x_{d}-x_{\mathrm{dd}}\right)\,\left(\frac{\frac{\psi _{\mathrm{1d},\mathrm{SG},D,3}\,\left(x_{\mathrm{dd}}-x_{\mathrm{ddd}}\right)}{x_{\mathrm{dd}}-x_{l}}-\psi _{d,\mathrm{SG},D,3}+\frac{\psi _{\mathrm{fd},\mathrm{SG},D,3}\,\left(x_{\mathrm{ddd}}-x_{l}\right)}{x_{\mathrm{dd}}-x_{l}}}{x_{\mathrm{ddd}}}-\frac{\left(x_{\mathrm{dd}}-x_{\mathrm{ddd}}\right)\,\left(\psi _{\mathrm{1d},\mathrm{SG},D,3}-\psi _{\mathrm{fd},\mathrm{SG},D,3}+\frac{\left(x_{\mathrm{dd}}-x_{l}\right)\,\left(\frac{\psi _{\mathrm{1d},\mathrm{SG},D,3}\,\left(x_{\mathrm{dd}}-x_{\mathrm{ddd}}\right)}{x_{\mathrm{dd}}-x_{l}}-\psi _{d,\mathrm{SG},D,3}+\frac{\psi _{\mathrm{fd},\mathrm{SG},D,3}\,\left(x_{\mathrm{ddd}}-x_{l}\right)}{x_{\mathrm{dd}}-x_{l}}\right)}{x_{\mathrm{ddd}}}\right)}{{\left(x_{\mathrm{dd}}-x_{l}\right)}^2}\right)}{T_{\mathrm{dd}}}$
      | Automatically generated on 2025-10-31 18:55:33 .
  State_E_fd_SG_D_3_0f771 : Inport
  State_psi_fd_SG_D_3_11ef0 : Inport  Port=2
  State_psi_1d_SG_D_3_aac28 : Inport  Port=3
  State_psi_fd_SG_D_3_d3ee5 : Inport  Port=4
  State_psi_1d_SG_D_3_07a55 : Inport  Port=5
  State_psi_d_SG_D_3_b2294 : Inport  Port=6
  State_psi_fd_SG_D_3_7f5a7 : Inport  Port=7
  State_psi_1d_SG_D_3_845cf : Inport  Port=8
  State_psi_d_SG_D_3_a29f0 : Inport  Port=9
  State_psi_fd_SG_D_3_791d9 : Inport  Port=10
  Add_93bb1 : Sum
  Add_a59e9 : Sum
  Constant_-1_4d6e5 : Constant  Value=-1
  Constant_-1_d5877 : Constant  Value=-1
  Constant_-1_e3027 : Constant  Value=-1
  Constant_2.0_94bb0 : Constant  Value=2.0
  Constant_T_dd_2cc39 : Constant  Value=T_dd
  Constant_x_d_adcf2 : Constant  Value=x_d
  Constant_x_dd_2269e : Constant  Value=x_dd
  Constant_x_dd_25836 : Constant  Value=x_dd
  Constant_x_dd_73a40 : Constant  Value=x_dd
  Constant_x_dd_7bf5f : Constant  Value=x_dd
  Constant_x_dd_a61d4 : Constant  Value=x_dd
  Constant_x_dd_b1fa4 : Constant  Value=x_dd
  Constant_x_dd_b2b0f : Constant  Value=x_dd
  Constant_x_dd_d64d4 : Constant  Value=x_dd
  Constant_x_dd_e6e75 : Constant  Value=x_dd
  Constant_x_dd_f9e13 : Constant  Value=x_dd
  Constant_x_ddd_2d8ec : Constant  Value=x_ddd
  Constant_x_ddd_af53f : Constant  Value=x_ddd
  Constant_x_ddd_c9406 : Constant  Value=x_ddd
  Constant_x_ddd_d0d04 : Constant  Value=x_ddd
  Constant_x_ddd_da24f : Constant  Value=x_ddd
  Constant_x_ddd_f5f5d : Constant  Value=x_ddd
  Constant_x_ddd_fd348 : Constant  Value=x_ddd
  Constant_x_l_4e98b : Constant  Value=x_l
  Constant_x_l_4eb73 : Constant  Value=x_l
  Constant_x_l_4ef81 : Constant  Value=x_l
  Constant_x_l_5cb71 : Constant  Value=x_l
  Constant_x_l_679d0 : Constant  Value=x_l
  Constant_x_l_68da3 : Constant  Value=x_l
  Constant_x_l_de405 : Constant  Value=x_l
  Constant_x_l_fe6ee : Constant  Value=x_l
  Divide_03a5a : Product  Inputs=*/
  Divide_19d0a : Product  Inputs=*/
  Divide_48e21 : Product  Inputs=*/
  Divide_5577c : Product  Inputs=*/
  Divide_aec10 : Product  Inputs=*/
  Divide_d3cda : Product  Inputs=*/
  Divide_da720 : Product  Inputs=*/
  Divide_dcad7 : Product  Inputs=*/
  Power_56e07 : Math  Operator=pow
  Product_0db3d : Product
  Product_11291 : Product
  Product_37c94 : Product
  Product_566b2 : Product
  Product_781b2 : Product
  Product_7bc2b : Product
  Product_ad3bd : Product
  Product_be086 : Product
  Product_c060a : Product
  Product_e759c : Product
  Subtract_2c7be : Sum  Inputs=+-
  Subtract_33530 : Sum  Inputs=+-
  Subtract_37b4f : Sum  Inputs=+-
  Subtract_3ae91 : Sum  Inputs=+-
  Subtract_453f0 : Sum  Inputs=+-
  Subtract_51322 : Sum  Inputs=+-
  Subtract_53502 : Sum  Inputs=+-
  Subtract_68f63 : Sum  Inputs=+-
  Subtract_730fb : Sum  Inputs=+-
  Subtract_78f66 : Sum  Inputs=+-
  Subtract_7ba3d : Sum  Inputs=+-
  Subtract_832e3 : Sum  Inputs=+-
  Subtract_8c66c : Sum  Inputs=+-
  Subtract_8dbfd : Sum  Inputs=+-
  Subtract_93d67 : Sum  Inputs=+-
  Subtract_98c20 : Sum  Inputs=+-
  Subtract_9ab3c : Sum  Inputs=+-
  Subtract_aa2ab : Sum  Inputs=+-
  Subtract_b2edf : Sum  Inputs=+-
  Blockout_d_psi_fd_SG_D_3_52489 : Outport
  wires:
  Product_11291/1 -> Divide_d3cda/1
  Constant_-1_4d6e5/1 -> Product_37c94/1
  Subtract_37b4f/1 -> Product_781b2/2
  State_psi_1d_SG_D_3_07a55/1 -> Product_37c94/2
  Constant_x_l_679d0/1 -> Subtract_2c7be/2
  Constant_x_dd_2269e/1 -> Subtract_37b4f/1
  Constant_x_ddd_da24f/1 -> Subtract_37b4f/2
  Product_37c94/1 -> Product_781b2/1
  Constant_x_dd_e6e75/1 -> Subtract_93d67/1
  Constant_x_l_de405/1 -> Subtract_93d67/2
  Constant_x_ddd_d0d04/1 -> Subtract_b2edf/2
  Constant_x_ddd_af53f/1 -> Subtract_3ae91/1
  Constant_x_l_4ef81/1 -> Subtract_3ae91/2
  Product_e759c/1 -> Product_be086/1
  Product_781b2/1 -> Divide_aec10/1
  Subtract_93d67/1 -> Divide_aec10/2
  State_psi_fd_SG_D_3_7f5a7/1 -> Product_566b2/1
  Constant_x_ddd_fd348/1 -> Subtract_2c7be/1
  Subtract_3ae91/1 -> Product_566b2/2
  Constant_x_dd_25836/1 -> Subtract_9ab3c/1
  Constant_-1_d5877/1 -> Product_e759c/1
  Constant_x_l_4eb73/1 -> Subtract_9ab3c/2
  Product_be086/1 -> Divide_03a5a/1
  Divide_aec10/1 -> Add_a59e9/1
  Product_ad3bd/1 -> Divide_48e21/1
  State_psi_d_SG_D_3_b2294/1 -> Add_a59e9/2
  State_psi_fd_SG_D_3_791d9/1 -> Product_ad3bd/1
  Product_566b2/1 -> Divide_da720/1
  Constant_x_dd_a61d4/1 -> Subtract_7ba3d/1
  Subtract_9ab3c/1 -> Divide_da720/2
  Constant_x_l_fe6ee/1 -> Subtract_aa2ab/2
  Constant_x_dd_b2b0f/1 -> Subtract_33530/1
  Subtract_453f0/1 -> Product_0db3d/2
  Constant_x_l_68da3/1 -> Subtract_33530/2
  Divide_03a5a/1 -> Add_93bb1/1
  Constant_x_ddd_2d8ec/1 -> Divide_d3cda/2
  Add_a59e9/1 -> Subtract_78f66/1
  Divide_da720/1 -> Subtract_78f66/2
  State_psi_1d_SG_D_3_845cf/1 -> Product_e759c/2
  Constant_x_l_5cb71/1 -> Subtract_7ba3d/2
  Constant_x_dd_d64d4/1 -> Subtract_b2edf/1
  Subtract_33530/1 -> Product_11291/1
  Add_93bb1/1 -> Subtract_730fb/1
  Subtract_78f66/1 -> Product_11291/2
  Subtract_b2edf/1 -> Product_be086/2
  Constant_x_dd_f9e13/1 -> Subtract_51322/1
  Constant_x_l_4e98b/1 -> Subtract_51322/2
  Subtract_2c7be/1 -> Product_ad3bd/2
  Constant_x_dd_b1fa4/1 -> Subtract_453f0/1
  Constant_x_ddd_c9406/1 -> Subtract_453f0/2
  Product_0db3d/1 -> Product_7bc2b/1
  State_psi_1d_SG_D_3_aac28/1 -> Subtract_832e3/1
  Subtract_51322/1 -> Divide_03a5a/2
  State_psi_fd_SG_D_3_d3ee5/1 -> Subtract_832e3/2
  Constant_-1_e3027/1 -> Product_0db3d/1
  Subtract_832e3/1 -> Subtract_68f63/1
  Divide_d3cda/1 -> Subtract_68f63/2
  Constant_x_dd_73a40/1 -> Subtract_aa2ab/1
  Divide_48e21/1 -> Subtract_730fb/2
  State_psi_d_SG_D_3_a29f0/1 -> Add_93bb1/2
  Subtract_7ba3d/1 -> Divide_48e21/2
  Subtract_68f63/1 -> Product_7bc2b/2
  Subtract_aa2ab/1 -> Power_56e07/1
  Constant_2.0_94bb0/1 -> Power_56e07/2
  Product_7bc2b/1 -> Divide_dcad7/1
  Subtract_8c66c/1 -> Product_c060a/2
  Power_56e07/1 -> Divide_dcad7/2
  Subtract_730fb/1 -> Divide_5577c/1
  Constant_x_ddd_f5f5d/1 -> Divide_5577c/2
  Constant_x_d_adcf2/1 -> Subtract_8dbfd/1
  Constant_x_dd_7bf5f/1 -> Subtract_8dbfd/2
  Divide_dcad7/1 -> Subtract_8c66c/1
  Divide_5577c/1 -> Subtract_8c66c/2
  State_E_fd_SG_D_3_0f771/1 -> Subtract_53502/1
  State_psi_fd_SG_D_3_11ef0/1 -> Subtract_53502/2
  Subtract_8dbfd/1 -> Product_c060a/1
  Subtract_53502/1 -> Subtract_98c20/1
  Product_c060a/1 -> Subtract_98c20/2
  Subtract_98c20/1 -> Divide_19d0a/1
  Constant_T_dd_2cc39/1 -> Divide_19d0a/2
  Divide_19d0a/1 -> Blockout_d_psi_fd_SG_D_3_52489/1
